simulink model "main"  (R2024b)
settings: Solver=FixedStepAuto  StartTime=0.0  StopTime=2.09  FixedStep=sample_time  RelTol=1e-3
values from neighbouring files (symbols this model uses):
  armTVC = [0 0 0.1064]    [matlab.mat]    (also in vars.m = [)
  att_control_rate = 0.01    [matlab.mat]
  c_d = 0.2    [matlab.mat]    (also in vars.m)
  contact =     [matlab.mat]
  g = 9.807    [matlab.mat]    (also in vars.m)
  initial_euler = [0 0 0]    [matlab.mat]
  m = 0.544    [matlab.mat]    (also in vars.m = 0.472)
  max_angle = 0.13962634016    [matlab.mat]
  rate_control_rate = 0.0025    [matlab.mat]
undefined symbols (not defined in the file or in its folder): fractalcoef, tf_tvc
libraries: sharedtransform x4, aerolibutil x3, sharedutil x3, simulink_extras x2, mspsensorlib x2, uavutilslib x1, shared6dof x1, simulink x1
settings Model: Creator=tommy  LastModifiedBy=tommy

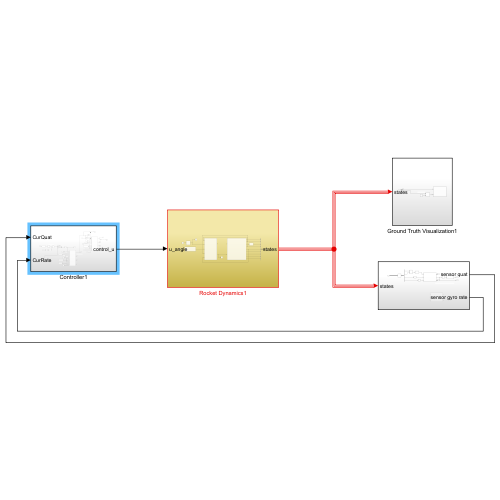
[thumbnail: Simulink's stored preview of the top-level diagram]
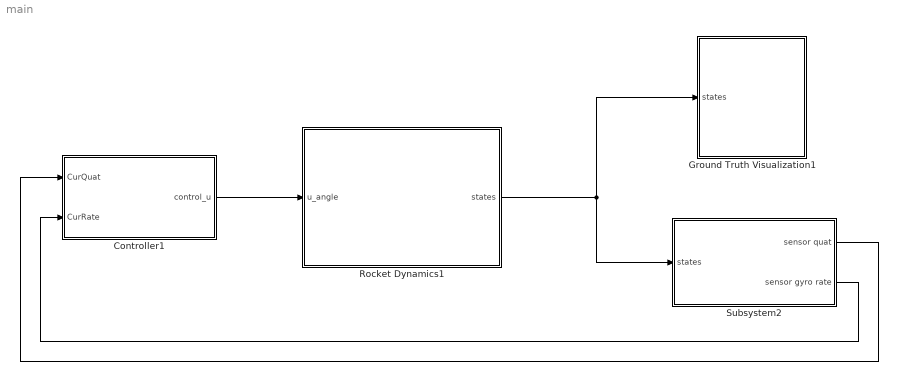
== system main ==
  Controller1 : Subsystem
  Ground Truth Visualization1 : Subsystem
  Rocket Dynamics1 : Subsystem
  Subsystem2 : Subsystem
  wires:
  Subsystem2/2(sensor gyro rate) -> Controller1/2(CurRate)
  Controller1/1(control_u) -> Rocket Dynamics1/1(u_angle)
  Subsystem2/1(sensor quat) -> Controller1/1(CurQuat)
  Rocket Dynamics1/1(states) -> Subsystem2/1(states), Ground Truth Visualization1/1(states)

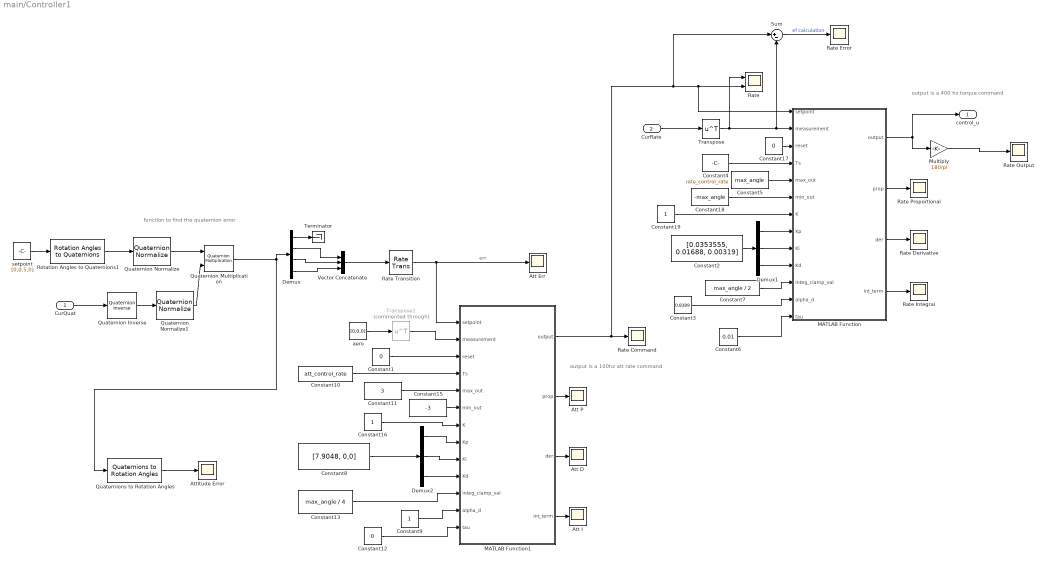
== system main/Controller1 ==
  note: output is a 100hz att rate command
  note: function to find the quaternion error
  note: output is a 400 hz torque command
  CurQuat : Inport
  CurRate : Inport  Port=2
  Att D : Scope
  Att Err : Scope
  Att I : Scope
  Att P : Scope
  Attitude Error : Scope
  Constant1 : Constant  Value=0
  Constant10 : Constant  Value=att_control_rate
  Constant11 : Constant  Value=3
  Constant12 : Constant  Value=0
  Constant13 : Constant  Value=max_angle / 4
  Constant15 : Constant  Value=-3
  Constant16 : Constant
  Constant17 : Constant  Value=0
  Constant18 : Constant  Value=-max_angle
  Constant19 : Constant
  Constant2 : Constant  Value=[0.0353555, 0.01688, 0.00319]
  Constant3 : Constant  Value=0.8389
  Constant4 : Constant  Value=rate_control_rate
  Constant5 : Constant  Value=max_angle
  Constant6 : Constant  Value=0.01
  Constant7 : Constant  Value=max_angle / 2
  Constant8 : Constant  Value=[7.9048, 0,0]
  Constant9 : Constant
  Demux : Demux
  Demux1 : Demux  Outputs=3
  Demux2 : Demux  Outputs=3
  MATLAB Function : MATLAB Function  TreatAsAtomicUnit=on  SystemSampleTime=rate_control_rate
  MATLAB Function1 : MATLAB Function  TreatAsAtomicUnit=on  SystemSampleTime=att_control_rate
  Multiply : Gain  Gain=180/pi
  Quaternion Inverse : aerolibutil/Quaternion Inverse
  Quaternion Multiplication : aerolibutil/Quaternion Multiplication
  Quaternion Normalize : sharedutil/Quaternion Normalize  aMode=aMode
  Quaternion Normalize1 : sharedutil/Quaternion Normalize  aMode=aMode
  Quaternions to Rotation Angles : sharedtransform/Quaternions to Rotation Angles  rotationOrder=XYZ  aMode=aMode
  Rate : Scope  NumInputPorts=2
  Rate Command : Scope
  Rate Derivative : Scope
  Rate Error : Scope
  Rate Integral : Scope
  Rate Output : Scope
  Rate Proportional : Scope
  Rate Transition : RateTransition  OutPortSampleTime=att_control_rate
  Rotation Angles to Quaternions1 : sharedtransform/Rotation Angles to Quaternions  rotationOrder=XYZ  aMode=aMode
  Sum : Sum  Inputs=|+-
  Terminator : Terminator
  Transpose : Math  Operator=transpose
  Transpose1 : Math  Commented=through  Operator=transpose
  Vector Concatenate : Concatenate  NumInputs=3
  aero : Constant  Value=[0,0,0]
  setpoint : Constant  Value=[0,0.5,0]
  control_u : Outport
  wires:
  setpoint/1 -> Rotation Angles to Quaternions1/1
  CurQuat/1 -> Quaternion Inverse/1
  Rotation Angles to Quaternions1/1 -> Quaternion Normalize/1
  Quaternion Inverse/1 -> Quaternion Normalize1/1
  Quaternion Normalize/1 -> Quaternion Multiplication/1
  Quaternion Normalize1/1 -> Quaternion Multiplication/2
  Demux/1 -> Terminator/1
  Quaternion Multiplication/1 -> Demux/1, Quaternions to Rotation Angles/1
  Demux/2 -> Vector Concatenate/1
  Demux/3 -> Vector Concatenate/2
  Demux/4 -> Vector Concatenate/3
  Quaternions to Rotation Angles/1 -> Attitude Error/1
  MATLAB Function/1(output) -> control_u/1, Multiply/1
  Vector Concatenate/1 -> Rate Transition/1
  CurRate/1 -> Transpose/1
  Sum/1 -> Rate Error/1  "ef calculation"
  Constant4/1 -> MATLAB Function/4(Ts)
  Transpose/1 -> MATLAB Function/2(measurement), Sum/2, Rate/1
  Constant6/1 -> MATLAB Function/13(tau)
  MATLAB Function/4(int_term) -> Rate Integral/1
  MATLAB Function/3(der) -> Rate Derivative/1
  MATLAB Function/2(prop) -> Rate Proportional/1
  Constant8/1 -> Demux2/1
  aero/1 -> Transpose1/1
  MATLAB Function1/2(prop) -> Att P/1
  MATLAB Function1/3(der) -> Att D/1
  MATLAB Function1/4(int_term) -> Att I/1
  Rate Transition/1 -> MATLAB Function1/1(setpoint), Att Err/1  "err"
  Demux2/1 -> MATLAB Function1/8(Kp)
  Demux2/2 -> MATLAB Function1/9(Ki)
  Demux2/3 -> MATLAB Function1/10(Kd)
  Constant13/1 -> MATLAB Function1/11(integ_clamp_val)
  Constant9/1 -> MATLAB Function1/12(alpha_d)
  Constant12/1 -> MATLAB Function1/13(tau)
  Constant10/1 -> MATLAB Function1/4(Ts)
  Constant1/1 -> MATLAB Function1/3(reset)
  Constant11/1 -> MATLAB Function1/5(max_out)
  Constant15/1 -> MATLAB Function1/6(min_out)
  Constant16/1 -> MATLAB Function1/7(K)
  Constant17/1 -> MATLAB Function/3(reset)
  Constant2/1 -> Demux1/1
  Constant3/1 -> MATLAB Function/12(alpha_d)
  Constant5/1 -> MATLAB Function/5(max_out)
  Constant18/1 -> MATLAB Function/6(min_out)
  Constant7/1 -> MATLAB Function/11(integ_clamp_val)
  Demux1/3 -> MATLAB Function/10(Kd)
  Demux1/2 -> MATLAB Function/9(Ki)
  Demux1/1 -> MATLAB Function/8(Kp)
  Constant19/1 -> MATLAB Function/7(K)
  Multiply/1 -> Rate Output/1
  Transpose1/1 -> MATLAB Function1/2(measurement)
  MATLAB Function1/1(output) -> Sum/1, MATLAB Function/1(setpoint), Rate/2, Rate Command/1

== system main/Ground Truth Visualization1 ==
  note: orient facing upwards
  states : Inport
  Bus Selector : BusSelector  OutputSignals=Xe,quat
  Constant : Constant  Value=eul2quat([0, pi/2, 0])  VectorParams1D=off
  Quaternion Multiplication : aerolibutil/Quaternion Multiplication
  UAV Animation1 : uavutilslib/UAV Animation  NumUAV=1  DynamicUAVConfig=off  UAVType=FixedWing  UAVSize=1  UAVColor=[1 0 0]  UAVTrajectoryAlpha=1  InertialZDirection=Down  RotationFormat=Quaternion  DrawMarkers=off  SampleTime=0.01
  wires:
  Constant/1 -> Quaternion Multiplication/2
  Quaternion Multiplication/1 -> UAV Animation1/2
  states/1 -> Bus Selector/1
  Bus Selector/1 -> UAV Animation1/1  "<Xe>"
  Bus Selector/2 -> Quaternion Multiplication/1  "<quat>"

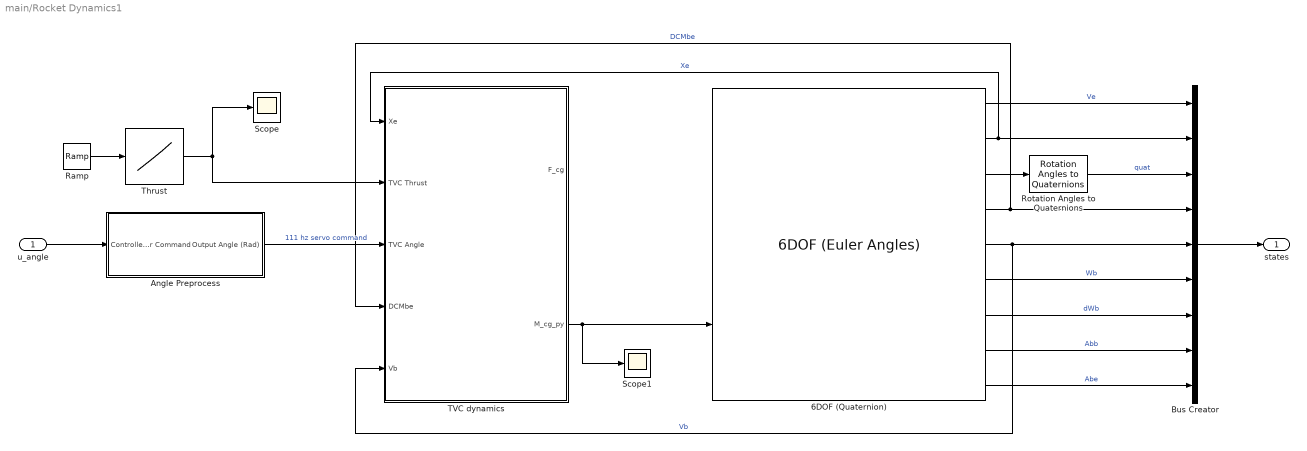
== system main/Rocket Dynamics1 ==
  u_angle : Inport
  6DOF (Quaternion) : shared6dof/6DOF (Euler Angles)  units=Metric (MKS)  mtype=Fixed  rep=Quaternion  xme_0=[0 0 0]  Vm_0=[0 0 0]  eul_0=initial_euler  pm_0=[0 0 0]  mass_0=m  mass_e=0.5  mass_f=2.0  inertia=inertia  inertia_e=eye(3)  inertia_f=2*eye(3)  k_quat=1  vre_flag=on  abi_flag=on  aMode=0  xme_statename=''  Vm_statename=''  eul_statename=''  quat_statename=''  pm_statename=''  mass_statename=''
  Angle Preprocess : Subsystem
  Bus Creator : BusCreator  Inputs=9
  Ramp : simulink/Sources/Ramp  slope=1  start=0  InitialOutput=0
  Rotation Angles to Quaternions : sharedtransform/Rotation Angles to Quaternions  rotationOrder=XYZ  aMode=aMode
  Scope : Scope
  Scope1 : Scope
  TVC dynamics : Subsystem
  Thrust : Lookup_n-D  NumberOfTableDimensions=1  BreakpointsForDimension1=[0;0.15;0.186;0.206;0.242;0.252;0.277;0.333;0.359;0.374;0.394;0.435;0.476;0.521;0.643;0.725;0.821;0.898;1.025;1.142;1.259;1.396;1.569;1.757;1.895;2.027;2.042;2.052;2.063;2.09;4;10]  Table=[0;1.371;1.92;3.387;5.587;7.422;8.705;13.474;15.858;16.592;18.609;21.544;24.661;26.44;21.72;20.432;19.511;18.958;18.219;18.032;17.844;17.472;17.282;17.275;17.086;17.816;12.494;8.457;4.97;0;0;0]  InterpMethod=Akima spline  InternalRulePriority=Speed  RndMeth=Simplest
  states : Outport
  wires:
  Bus Creator/1 -> states/1
  TVC dynamics/2(M_cg_py) -> Scope1/1, 6DOF (Quaternion)/2
  6DOF (Quaternion)/7 -> Bus Creator/7  "dWb"
  Angle Preprocess/1(Output Angle (Rad)) -> TVC dynamics/3(TVC Angle)  "111 hz servo command"
  6DOF (Quaternion)/3 -> Rotation Angles to Quaternions/1
  6DOF (Quaternion)/6 -> Bus Creator/6  "Wb"
  6DOF (Quaternion)/9 -> Bus Creator/9  "Abe"
  6DOF (Quaternion)/5 -> TVC dynamics/5(Vb), Bus Creator/5  "Vb"
  6DOF (Quaternion)/1 -> Bus Creator/1  "Ve"
  u_angle/1 -> Angle Preprocess/1(Controller Command)
  6DOF (Quaternion)/4 -> TVC dynamics/4(DCMbe), Bus Creator/4  "DCMbe"
  6DOF (Quaternion)/2 -> TVC dynamics/1(Xe), Bus Creator/2  "Xe"
  Rotation Angles to Quaternions/1 -> Bus Creator/3  "quat"
  Thrust/1 -> TVC dynamics/2(TVC Thrust), Scope/1
  Ramp/1 -> Thrust/1
  6DOF (Quaternion)/8 -> Bus Creator/8  "Abb"

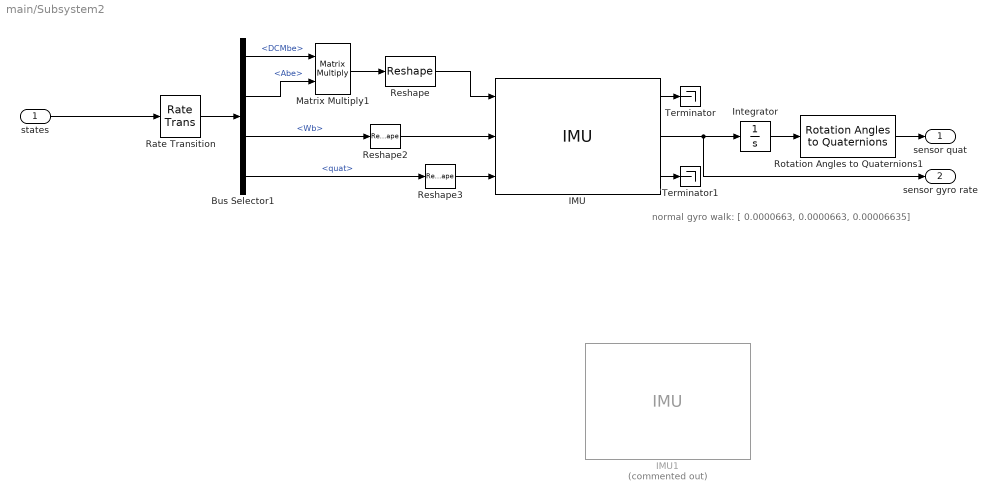
== system main/Subsystem2 ==
  note: normal gyro walk: [ 0.0000663, 0.0000663, 0.00006635]
  states : Inport
  Bus Selector1 : BusSelector  OutputSignals=DCMbe,Abe,Wb,quat
  IMU : mspsensorlib/IMU  DispRefFrame=NED  TemperaturePort=off  Temperature=0  MagneticFieldPort=off  MagneticFieldNED=[ 27.5550, -2.4169, -16.0849 ]  MagneticFieldENU=[ -2.4169, 27.5550, 16.0849 ]  SeedDouble=67  SimulateUsing=Interpreted execution  AccelParamsMeasurementRange=Inf  AccelParamsResolution=0  AccelParamsConstantBias=[ 0, 0, 0 ]  AccelParamsAxesMisalignment=[ 1, 0, 0; 0, 1, 0; 0, 0, 1 ]  AccelParamsNoiseDensity=[ 0, 0, 0 ]  AccelParamsBiasInstability=[ 0, 0, 0 ]  AccelParamsBiasInstabilityNumerator=fractalcoef().Numerator  AccelParamsBiasInstabilityDenominator=fractalcoef().Denominator  AccelParamsRandomWalk=[ 0, 0, 0 ]  AccelParamsNoiseType=double-sided  AccelParamsTemperatureBias=[ 0, 0, 0 ]  AccelParamsTemperatureScaleFactor=[ 0, 0, 0 ]  GyroParamsMeasurementRange=Inf  GyroParamsResolution=0  GyroParamsConstantBias=[ 0, 0, 0 ]  GyroParamsAxesMisalignment=[ 100, 0, 0; 0, 100, 0; 0, 0, 100 ]  GyroParamsAccelerationBias=[ 0, 0, 0 ]  GyroParamsNoiseDensity=[0, 0, 0]  GyroParamsBiasInstability=[ 0, 0, 0 ]  GyroParamsBiasInstabilityNumerator=fractalcoef().Numerator  GyroParamsBiasInstabilityDenominator=fractalcoef().Denominator  GyroParamsRandomWalk=[ 0, 0, 0 ]  GyroParamsNoiseType=double-sided  GyroParamsTemperatureBias=[ 0, 0, 0 ]  GyroParamsTemperatureScaleFactor=[ 0, 0, 0 ]  MagParamsMeasurementRange=Inf  MagParamsResolution=0  MagParamsConstantBias=[ 0, 0, 0 ]  MagParamsAxesMisalignment=[ 100, 0, 0; 0, 100, 0; 0, 0, 100 ]  MagParamsNoiseDensity=[ 0, 0, 0 ]  MagParamsBiasInstability=[ 0, 0, 0 ]  MagParamsBiasInstabilityNumerator=fractalcoef().Numerator  MagParamsBiasInstabilityDenominator=fractalcoef().Denominator  MagParamsRandomWalk=[ 0, 0, 0 ]  MagParamsNoiseType=double-sided  MagParamsTemperatureBias=[ 0, 0, 0 ]  MagParamsTemperatureScaleFactor=[ 0, 0, 0 ]
  IMU1 : mspsensorlib/IMU  Commented=on  DispRefFrame=NED  TemperaturePort=off  Temperature=0  MagneticFieldPort=off  MagneticFieldNED=[ 27.5550, -2.4169, -16.0849 ]  MagneticFieldENU=[ -2.4169, 27.5550, 16.0849 ]  SeedDouble=67  SimulateUsing=Interpreted execution  AccelParamsMeasurementRange=Inf  AccelParamsResolution=0  AccelParamsConstantBias=[ 0, 0, 0 ]  AccelParamsAxesMisalignment=[ 1, 0, 0; 0, 1, 0; 0, 0, 1 ]  AccelParamsNoiseDensity=[ 0, 0, 0 ]  AccelParamsBiasInstability=[ 0, 0, 0 ]  AccelParamsBiasInstabilityNumerator=fractalcoef().Numerator  AccelParamsBiasInstabilityDenominator=fractalcoef().Denominator  AccelParamsRandomWalk=[ 0, 0, 0 ]  AccelParamsNoiseType=double-sided  AccelParamsTemperatureBias=[ 0, 0, 0 ]  AccelParamsTemperatureScaleFactor=[ 0, 0, 0 ]  GyroParamsMeasurementRange=Inf  GyroParamsResolution=0  GyroParamsConstantBias=[ 0, 0, 0 ]  GyroParamsAxesMisalignment=[ 100, 0, 0; 0, 100, 0; 0, 0, 100 ]  GyroParamsAccelerationBias=[ 0, 0, 0 ]  GyroParamsNoiseDensity=[ 0.0000663, 0.0000663, 0.00006635]  GyroParamsBiasInstability=[ 0, 0, 0 ]  GyroParamsBiasInstabilityNumerator=fractalcoef().Numerator  GyroParamsBiasInstabilityDenominator=fractalcoef().Denominator  GyroParamsRandomWalk=[ 0, 0, 0 ]  GyroParamsNoiseType=double-sided  GyroParamsTemperatureBias=[ 0, 0, 0 ]  GyroParamsTemperatureScaleFactor=[ 0, 0, 0 ]  MagParamsMeasurementRange=Inf  MagParamsResolution=0  MagParamsConstantBias=[ 0, 0, 0 ]  MagParamsAxesMisalignment=[ 100, 0, 0; 0, 100, 0; 0, 0, 100 ]  MagParamsNoiseDensity=[ 0, 0, 0 ]  MagParamsBiasInstability=[ 0, 0, 0 ]  MagParamsBiasInstabilityNumerator=fractalcoef().Numerator  MagParamsBiasInstabilityDenominator=fractalcoef().Denominator  MagParamsRandomWalk=[ 0, 0, 0 ]  MagParamsNoiseType=double-sided  MagParamsTemperatureBias=[ 0, 0, 0 ]  MagParamsTemperatureScaleFactor=[ 0, 0, 0 ]
  Integrator : Integrator  InitialCondition=initial_euler
  Matrix Multiply1 : Product  Multiplication=Matrix(*)
  Rate Transition : RateTransition  OutPortSampleTime=sample_time
  Reshape : Reshape  OutputDimensionality=Row vector (2-D)
  Reshape2 : Reshape  OutputDimensionality=Row vector (2-D)
  Reshape3 : Reshape  OutputDimensionality=Row vector (2-D)
  Rotation Angles to Quaternions1 : sharedtransform/Rotation Angles to Quaternions  rotationOrder=XYZ  aMode=aMode
  Terminator : Terminator
  Terminator1 : Terminator
  sensor quat : Outport
  sensor gyro rate : Outport  Port=2
  wires:
  Reshape2/1 -> IMU/2
  IMU/2 -> Integrator/1, sensor gyro rate/1
  Matrix Multiply1/1 -> Reshape/1
  Reshape/1 -> IMU/1
  Integrator/1 -> Rotation Angles to Quaternions1/1
  Reshape3/1 -> IMU/3
  Bus Selector1/4 -> Reshape3/1  "<quat>"
  Bus Selector1/3 -> Reshape2/1  "<Wb>"
  Rotation Angles to Quaternions1/1 -> sensor quat/1
  states/1 -> Rate Transition/1
  Rate Transition/1 -> Bus Selector1/1
  IMU/1 -> Terminator/1
  IMU/3 -> Terminator1/1
  Bus Selector1/1 -> Matrix Multiply1/1  "<DCMbe>"
  Bus Selector1/2 -> Matrix Multiply1/2  "<Abe>"

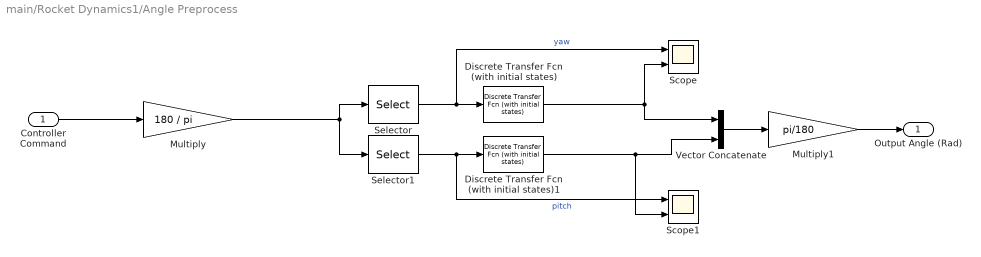
== system main/Rocket Dynamics1/Angle Preprocess ==
  Controller Command : Inport
  Discrete Transfer Fcn (with initial states) : simulink_extras/Additional Discrete/Discrete Transfer Fcn (with initial states)  N=tf_tvc.Numerator  D=tf_tvc.Denominator  X0=[1]  TS=tf_tvc.Ts
  Discrete Transfer Fcn (with initial states)1 : simulink_extras/Additional Discrete/Discrete Transfer Fcn (with initial states)  N=tf_tvc.Numerator  D=tf_tvc.Denominator  X0=[1]  TS=tf_tvc.Ts
  Multiply : Gain  Gain=180 / pi
  Multiply1 : Gain  Gain=pi/180
  Scope : Scope  NumInputPorts=2
  Scope1 : Scope  NumInputPorts=2
  Selector : Selector  InputPortWidth=3  IndexOptions=Index vector (dialog)  Indices=[1]  OutputSizes=1
  Selector1 : Selector  InputPortWidth=3  IndexOptions=Index vector (dialog)  Indices=[2]  OutputSizes=1
  Vector Concatenate : Concatenate
  Output Angle (Rad) : Outport
  wires:
  Vector Concatenate/1 -> Multiply1/1
  Controller Command/1 -> Multiply/1
  Selector/1 -> Discrete Transfer Fcn (with initial states)/1, Scope/1  "yaw"
  Multiply1/1 -> Output Angle (Rad)/1
  Discrete Transfer Fcn (with initial states)/1 -> Vector Concatenate/1, Scope/2
  Discrete Transfer Fcn (with initial states)1/1 -> Scope1/2, Vector Concatenate/2
  Multiply/1 -> Selector1/1, Selector/1
  Selector1/1 -> Scope1/1, Discrete Transfer Fcn (with initial states)1/1  "pitch"

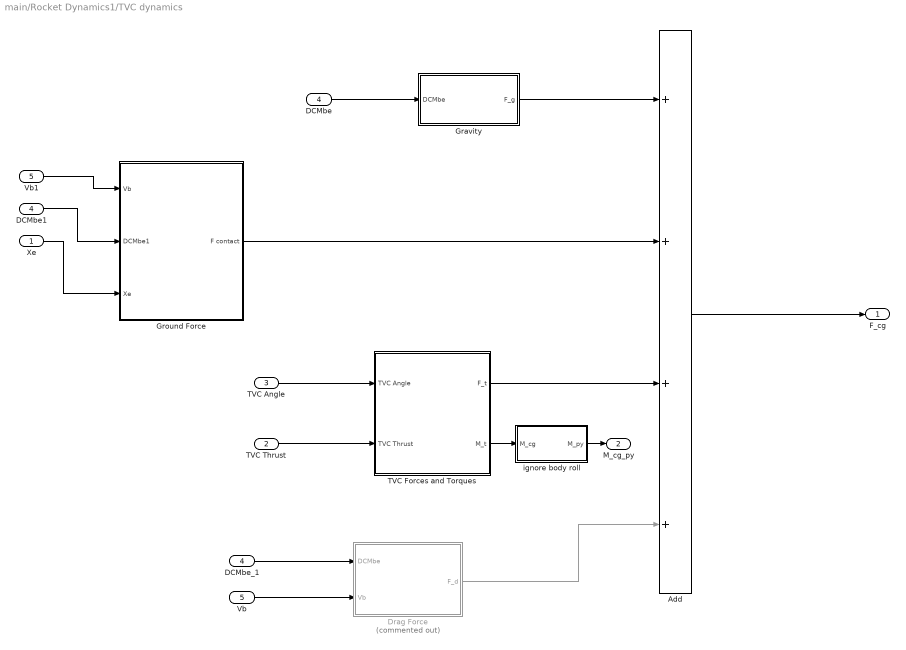
== system main/Rocket Dynamics1/TVC dynamics ==
  Xe : Inport
  TVC Thrust : Inport  Port=2
  TVC Angle : Inport  Port=3
  DCMbe : Inport  Port=4
  Vb : Inport  Port=5
  Add : Sum  Inputs=++++
  DCMbe1 : InportShadow  Port=4
  DCMbe_1 : InportShadow  Port=4
  Drag Force : Subsystem  Commented=on
  Gravity : Subsystem
  Ground Force : Subsystem
  TVC Forces and Torques : Subsystem
  Vb1 : InportShadow  Port=5
  "ignore body roll " : Subsystem
  F_cg : Outport
  M_cg_py : Outport  Port=2
  wires:
  Add/1 -> F_cg/1
  DCMbe_1/1 -> Drag Force/1(DCMbe)
  TVC Forces and Torques/1(F_t) -> Add/3
  Vb/1 -> Drag Force/2(Vb)
  Gravity/1(F_g) -> Add/1
  TVC Thrust/1 -> TVC Forces and Torques/2(TVC Thrust)
  TVC Forces and Torques/2(M_t) -> "ignore body roll "/1(M_cg)
  DCMbe/1 -> Gravity/1(DCMbe)
  TVC Angle/1 -> TVC Forces and Torques/1(TVC Angle)
  Drag Force/1(F_d) -> Add/4
  DCMbe1/1 -> Ground Force/2(DCMbe1)
  Xe/1 -> Ground Force/3(Xe)
  Ground Force/1(F contact) -> Add/2
  Vb1/1 -> Ground Force/1(Vb)
  "ignore body roll "/1(M_py) -> M_cg_py/1

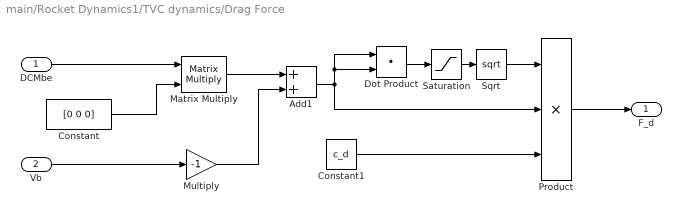
== system main/Rocket Dynamics1/TVC dynamics/Drag Force ==
  DCMbe : Inport
  Vb : Inport  Port=2
  Add1 : Sum
  Constant : Constant  Value=[0 0 0]
  Constant1 : Constant  Value=c_d
  Dot Product : DotProduct  OutDataTypeStr=Inherit: Inherit via internal rule
  Matrix Multiply : Product  Multiplication=Matrix(*)
  Multiply : Gain  Gain=-1
  Product : Product  Inputs=3
  Saturation : Saturate  UpperLimit=inf  LowerLimit=0.00001
  Sqrt : Sqrt
  F_d : Outport
  wires:
  Dot Product/1 -> Saturation/1
  Multiply/1 -> Add1/2
  Constant/1 -> Matrix Multiply/2
  Matrix Multiply/1 -> Add1/1
  Add1/1 -> Product/2, Dot Product/1, Dot Product/2
  Vb/1 -> Multiply/1
  DCMbe/1 -> Matrix Multiply/1
  Sqrt/1 -> Product/1
  Saturation/1 -> Sqrt/1
  Product/1 -> F_d/1
  Constant1/1 -> Product/3

== system main/Rocket Dynamics1/TVC dynamics/Gravity ==
  DCMbe : Inport
  Constant : Constant  Value=[0 0 g]
  Matrix Multiply : Product  Multiplication=Matrix(*)
  Multiply : Gain  Gain=m
  F_g : Outport
  wires:
  Multiply/1 -> Matrix Multiply/2
  DCMbe/1 -> Matrix Multiply/1
  Constant/1 -> Multiply/1
  Matrix Multiply/1 -> F_g/1

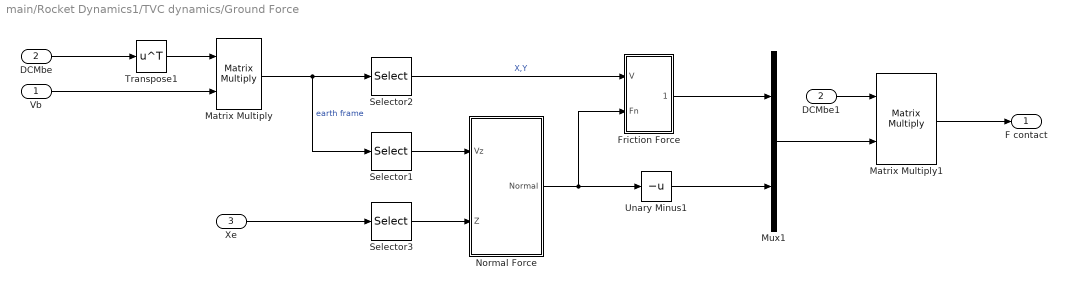
== system main/Rocket Dynamics1/TVC dynamics/Ground Force ==
  Vb : Inport
  DCMbe1 : Inport  Port=2
  Xe : Inport  Port=3
  DCMbe : InportShadow  Port=2
  Friction Force : Subsystem
  Matrix Multiply : Product  Multiplication=Matrix(*)
  Matrix Multiply1 : Product  Multiplication=Matrix(*)
  Mux1 : Mux  Inputs=2
  Normal Force : Subsystem
  Selector1 : Selector  InputPortWidth=3  IndexOptions=Index vector (dialog)  Indices=[3]  OutputSizes=1
  Selector2 : Selector  InputPortWidth=3  IndexOptions=Index vector (dialog)  Indices=[1,2]  OutputSizes=1
  Selector3 : Selector  InputPortWidth=3  IndexOptions=Index vector (dialog)  Indices=[3]  OutputSizes=1
  Transpose1 : Math  Operator=transpose
  Unary Minus1 : UnaryMinus
  F contact : Outport
  wires:
  Matrix Multiply1/1 -> F contact/1
  Friction Force/1(Friction) -> Mux1/1
  Xe/1 -> Selector3/1
  Vb/1 -> Matrix Multiply/2
  Selector3/1 -> Normal Force/2(Z)
  Matrix Multiply/1 -> Selector1/1, Selector2/1  "earth frame"
  Mux1/1 -> Matrix Multiply1/2
  Selector2/1 -> Friction Force/1(V)  "X,Y"
  Selector1/1 -> Normal Force/1(Vz)
  DCMbe1/1 -> Matrix Multiply1/1
  DCMbe/1 -> Transpose1/1
  Transpose1/1 -> Matrix Multiply/1
  Unary Minus1/1 -> Mux1/2
  Normal Force/1(Normal) -> Unary Minus1/1, Friction Force/2(Fn)

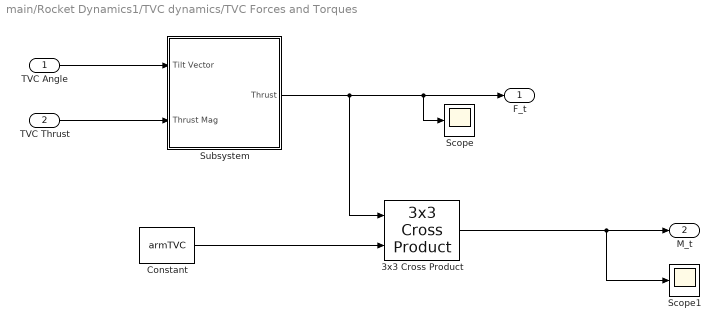
== system main/Rocket Dynamics1/TVC dynamics/TVC Forces and Torques ==
  TVC Angle : Inport
  TVC Thrust : Inport  Port=2
  3x3 Cross Product : sharedutil/3x3 Cross Product  aMode=aMode
  Constant : Constant  Value=armTVC
  Scope : Scope
  Scope1 : Scope
  Subsystem : Subsystem
  F_t : Outport
  M_t : Outport  Port=2
  wires:
  TVC Angle/1 -> Subsystem/1(Tilt Vector)
  TVC Thrust/1 -> Subsystem/2(Thrust Mag)
  Subsystem/1(Thrust) -> 3x3 Cross Product/1, Scope/1, F_t/1
  Constant/1 -> 3x3 Cross Product/2
  3x3 Cross Product/1 -> Scope1/1, M_t/1

== system main/Rocket Dynamics1/TVC dynamics/ignore body roll  ==
  M_cg : Inport
  Constant1 : Constant  Value=[1, 1, 0]
  Matrix Multiply : Product
  M_py : Outport
  wires:
  Constant1/1 -> Matrix Multiply/1
  Matrix Multiply/1 -> M_py/1
  M_cg/1 -> Matrix Multiply/2

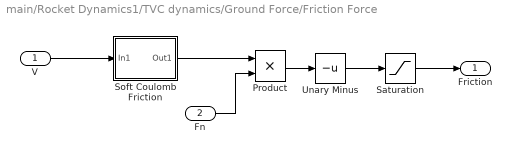
== system main/Rocket Dynamics1/TVC dynamics/Ground Force/Friction Force ==
  V : Inport
  Fn : Inport  Port=2
  Product : Product
  Saturation : Saturate  UpperLimit=contact.translation.maxFriction  LowerLimit=-contact.translation.maxFriction
  Soft Coulomb Friction : Subsystem
  Unary Minus : UnaryMinus
  Friction : Outport
  wires:
  Fn/1 -> Product/2
  Soft Coulomb Friction/1(Out1) -> Product/1
  Product/1 -> Unary Minus/1
  V/1 -> Soft Coulomb Friction/1(In1)
  Unary Minus/1 -> Saturation/1
  Saturation/1 -> Friction/1

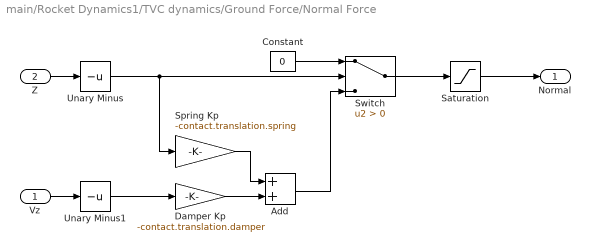
== system main/Rocket Dynamics1/TVC dynamics/Ground Force/Normal Force ==
  Vz : Inport
  Z : Inport  Port=2
  Add : Sum
  Constant : Constant  Value=0
  Damper Kp : Gain  Gain=-contact.translation.damper
  Saturation : Saturate  UpperLimit=contact.translation.maxNormal  LowerLimit=0
  Spring Kp : Gain  Gain=-contact.translation.spring
  Switch : Switch  Criteria=u2 > Threshold  SaturateOnIntegerOverflow=off  InputSameDT=off
  Unary Minus : UnaryMinus
  Unary Minus1 : UnaryMinus
  Normal : Outport
  wires:
  Constant/1 -> Switch/1
  Z/1 -> Unary Minus/1
  Switch/1 -> Saturation/1
  Damper Kp/1 -> Add/2
  Add/1 -> Switch/3
  Spring Kp/1 -> Add/1
  Vz/1 -> Unary Minus1/1
  Saturation/1 -> Normal/1
  Unary Minus/1 -> Spring Kp/1, Switch/2
  Unary Minus1/1 -> Damper Kp/1

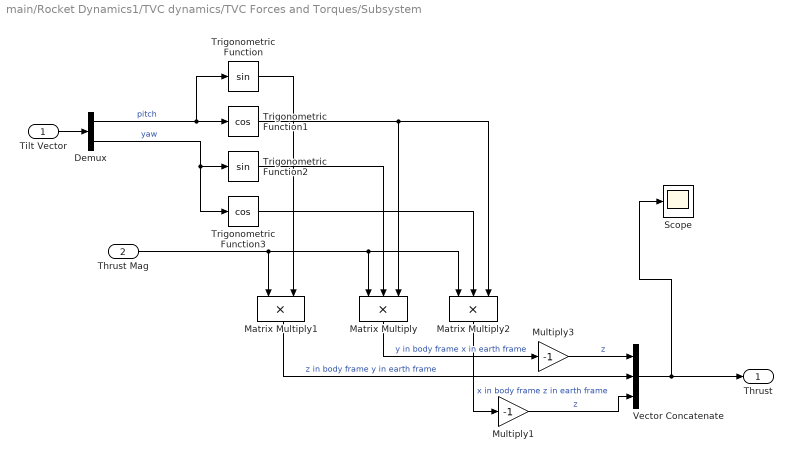
== system main/Rocket Dynamics1/TVC dynamics/TVC Forces and Torques/Subsystem ==
  Tilt Vector : Inport
  Thrust Mag : Inport  Port=2
  Demux : Demux  Outputs=2
  Matrix Multiply : Product  Inputs=3
  Matrix Multiply1 : Product
  Matrix Multiply2 : Product  Inputs=3
  Multiply1 : Gain  Gain=-1
  Multiply3 : Gain  Gain=-1
  Scope : Scope
  Trigonometric Function : Trigonometry
  Trigonometric Function1 : Trigonometry  Operator=cos
  Trigonometric Function2 : Trigonometry
  Trigonometric Function3 : Trigonometry  Operator=cos
  Vector Concatenate : Concatenate  NumInputs=3
  Thrust : Outport
  wires:
  Trigonometric Function2/1 -> Matrix Multiply/2
  Demux/2 -> Trigonometric Function3/1, Trigonometric Function2/1  "yaw"
  Matrix Multiply1/1 -> Vector Concatenate/2  "z in body frame y in earth frame"
  Tilt Vector/1 -> Demux/1
  Trigonometric Function1/1 -> Matrix Multiply/3, Matrix Multiply2/3
  Demux/1 -> Trigonometric Function/1, Trigonometric Function1/1  "pitch"
  Trigonometric Function3/1 -> Matrix Multiply2/2
  Thrust Mag/1 -> Matrix Multiply2/1, Matrix Multiply/1, Matrix Multiply1/1
  Vector Concatenate/1 -> Scope/1, Thrust/1
  Trigonometric Function/1 -> Matrix Multiply1/2
  Matrix Multiply2/1 -> Multiply1/1  "x in body frame z in earth frame"
  Multiply1/1 -> Vector Concatenate/3  "z"
  Multiply3/1 -> Vector Concatenate/1  "z"
  Matrix Multiply/1 -> Multiply3/1  "y in body frame x in earth frame"

== system main/Rocket Dynamics1/TVC dynamics/Ground Force/Friction Force/Soft Coulomb Friction ==
  note: Pennestrì, E., Rossi, V., Salvini, P. et al. Review and comparison of dry friction force models. Nonlinear Dyn 83, 1785–1801 (2016). https://doi.org/10.1007/s11071-015-2485-3
  In1 : Inport
  Tanh : Trigonometry  Operator=tanh
  friction coefficient : Gain  Gain=contact.translation.friction
  vd : Gain  Gain=1/contact.translation.vd
  Out1 : Outport
  wires:
  In1/1 -> vd/1
  vd/1 -> Tanh/1
  Tanh/1 -> friction coefficient/1
  friction coefficient/1 -> Out1/1

== matlab function main/Controller1/MATLAB Function ==
  data: setpoint input; output output; prop output; der output; measurement input; reset input; Ts input; max_out input; min_out input; K input; Kp input; Ki input; Kd input; integ_clamp_val input; alpha_d input; tau input; int_term output
function [output, prop, der, int_term] = PID_SF_Matlab(setpoint, measurement, reset, Ts, max_out, min_out, K, Kp, Ki, Kd, integ_clamp_val, alpha_d, tau)
% PID_SF_Matlab: A standard form PID controller translated from a C++ implementation.
%
% This controller features several enhancements over a basic PID:
%   - Derivative on measurement: Prevents "derivative kick" on setpoint changes.
%   - Integral clamping: Directly limits the integral term to prevent excessive windup.
%   - Conditional integration (anti-windup): Stops integration when the output is saturated.
%   - Output filtering: Smooths the final control signal using a low-pass filter.
%
% It is designed to be a "plug-and-play" replacement for the original PID_Simulink
% function and supports N-dimensional vector inputs.
%
% Inputs:
%   setpoint        - Desired setpoint (e.g., 3x1 vector).
%   measurement     - Measured process variable (e.g., 3x1 vector).
%   reset           - Boolean flag (1 or true) to reset the controller's internal states.
%   Ts              - Sampling time in seconds (scalar).
%   max_out         - Maximum output value (scalar).
%   min_out         - Minimum output value (scalar).
%   K               - Overall system gain (scalar).
%   Kp              - Proportional gain (scalar).
%   Ki              - Integral gain (scalar).
%   Kd              - Derivative gain (scalar).
%   integ_clamp_val - User-friendly absolute integral clamp value (e.g., 500 for a servo).
%   alpha_d         - Smoothing factor for the derivative term (0 to 1). A smaller value means more smoothing.
%   tau             - Time constant for the output low-pass filter in seconds (scalar). Larger tau means more smoothing.
%
% Outputs:
%   output          - The final, filtered PID control signal (same dimensions as input).
%   prop            - The proportional component of the output.
%   der             - The derivative component of the output.
%   int_term        - The integral component of the output.

% Declare persistent variables to hold the controller's state between calls.
persistent integral_state prev_meas derivative_state old_output_filtered

% Initialize states to zero on the first call or when the reset flag is true.
% This corrected block ensures persistent variables are only checked with isempty
% before their first assignment.
if isempty(integral_state) || reset
    vec_size = size(setpoint);
    integral_state = zeros(vec_size);
    prev_meas = zeros(vec_size);
    derivative_state = zeros(vec_size);
    old_output_filtered = zeros(vec_size);
end

% --- Parameter Pre-calculation (for efficiency, mirrors C++ setup) ---

% Add robustness against invalid sampling time.
if Ts <= 0
    Ts = 1e-6; % Use a very small number to prevent division by zero.
end

% Pre-multiply/divide gains by Ts to save computation in the main loop.
ki_Ts = Ki * Ts;
kd_Ts = Kd / Ts;

% Scale the user-provided integral clamp value based on the system gains.
% This translates the desired absolute clamp into the correct internal value.
if (K * ki_Ts > 0)
    integ_clamp_scaled = integ_clamp_val / (K * ki_Ts);
else
    integ_clamp_scaled = 0;
end

% Calculate the output low-pass filter coefficient from the time constant.
if (Ts + tau) > 1e-6
    alpha_lpf = Ts / (Ts + tau);
else
    alpha_lpf = 1.0;
end

% --- Core PID Logic ---

% 1. Calculate the error.
error = setpoint - measurement;

% 2. Calculate the filtered derivative on the measurement, not the error.
% This is a low-pass filter on the rate of change of the measurement.
derivative_state = alpha_d .* (measurement - prev_meas) + (1 - alpha_d) .* derivative_state;

% 3. Calculate the individual P, I, and D components for the output signal.
prop     = K .* Kp .* error;
int_term = K .* ki_Ts .* integral_state;
der      = -K .* kd_Ts .* derivative_state; % Note the negative sign.

% 4. Sum the components to get the preliminary, unfiltered output.
output_pre_clamp = prop + int_term + der;

% 5. Apply output saturation and conditional integration (anti-windup).
% This loop is necessary to handle vector inputs correctly.
output = output_pre_clamp;
for i = 1:numel(output)
    if output(i) > max_out
        output(i) = max_out;
    elseif output(i) < min_out
        output(i) = min_out;
    else
        % ONLY update the integral if the output is NOT saturated.
        integral_state(i) = integral_state(i) + error(i);
    end
end

% 6. Apply the direct clamp on the integral state itself.
for i = 1:numel(integral_state)
    if integral_state(i) > integ_clamp_scaled
        integral_state(i) = integ_clamp_scaled;
    elseif integral_state(i) < -integ_clamp_scaled
        integral_state(i) = -integ_clamp_scaled;
    end
end

% 8. Update persistent states for the next function call.
prev_meas = measurement;
old_output_filtered = output;

end

== matlab function main/Controller1/MATLAB Function1 ==
  data: setpoint input; output output; prop output; der output; measurement input; reset input; Ts input; max_out input; min_out input; K input; Kp input; Ki input; Kd input; integ_clamp_val input; alpha_d input; tau input; int_term output
function [output, prop, der, int_term] = PID_SF_Matlab(setpoint, measurement, reset, Ts, max_out, min_out, K, Kp, Ki, Kd, integ_clamp_val, alpha_d, tau)
% PID_SF_Matlab: A standard form PID controller translated from a C++ implementation.
%
% This controller features several enhancements over a basic PID:
%   - Derivative on measurement: Prevents "derivative kick" on setpoint changes.
%   - Integral clamping: Directly limits the integral term to prevent excessive windup.
%   - Conditional integration (anti-windup): Stops integration when the output is saturated.
%   - Output filtering: Smooths the final control signal using a low-pass filter.
%
% It is designed to be a "plug-and-play" replacement for the original PID_Simulink
% function and supports N-dimensional vector inputs.
%
% Inputs:
%   setpoint        - Desired setpoint (e.g., 3x1 vector).
%   measurement     - Measured process variable (e.g., 3x1 vector).
%   reset           - Boolean flag (1 or true) to reset the controller's internal states.
%   Ts              - Sampling time in seconds (scalar).
%   max_out         - Maximum output value (scalar).
%   min_out         - Minimum output value (scalar).
%   K               - Overall system gain (scalar).
%   Kp              - Proportional gain (scalar).
%   Ki              - Integral gain (scalar).
%   Kd              - Derivative gain (scalar).
%   integ_clamp_val - User-friendly absolute integral clamp value (e.g., 500 for a servo).
%   alpha_d         - Smoothing factor for the derivative term (0 to 1). A smaller value means more smoothing.
%   tau             - Time constant for the output low-pass filter in seconds (scalar). Larger tau means more smoothing.
%
% Outputs:
%   output          - The final, filtered PID control signal (same dimensions as input).
%   prop            - The proportional component of the output.
%   der             - The derivative component of the output.
%   int_term        - The integral component of the output.

% Declare persistent variables to hold the controller's state between calls.
persistent integral_state prev_meas derivative_state old_output_filtered

% Initialize states to zero on the first call or when the reset flag is true.
% This corrected block ensures persistent variables are only checked with isempty
% before their first assignment.
if isempty(integral_state) || reset
    vec_size = size(setpoint);
    integral_state = zeros(vec_size);
    prev_meas = zeros(vec_size);
    derivative_state = zeros(vec_size);
    old_output_filtered = zeros(vec_size);
end

% --- Parameter Pre-calculation (for efficiency, mirrors C++ setup) ---

% Add robustness against invalid sampling time.
if Ts <= 0
    Ts = 1e-6; % Use a very small number to prevent division by zero.
end

% Pre-multiply/divide gains by Ts to save computation in the main loop.
ki_Ts = Ki * Ts;
kd_Ts = Kd / Ts;

% Scale the user-provided integral clamp value based on the system gains.
% This translates the desired absolute clamp into the correct internal value.
if (K * ki_Ts > 0)
    integ_clamp_scaled = integ_clamp_val / (K * ki_Ts);
else
    integ_clamp_scaled = 0;
end

% Calculate the output low-pass filter coefficient from the time constant.
if (Ts + tau) > 1e-6
    alpha_lpf = Ts / (Ts + tau);
else
    alpha_lpf = 1.0;
end

% --- Core PID Logic ---

% 1. Calculate the error.
error = setpoint - measurement;

% 2. Calculate the filtered derivative on the measurement, not the error.
% This is a low-pass filter on the rate of change of the measurement.
derivative_state = alpha_d .* (measurement - prev_meas) + (1 - alpha_d) .* derivative_state;

% 3. Calculate the individual P, I, and D components for the output signal.
prop     = K .* Kp .* error;
int_term = K .* ki_Ts .* integral_state;
der      = -K .* kd_Ts .* derivative_state; % Note the negative sign.

% 4. Sum the components to get the preliminary, unfiltered output.
output_pre_clamp = prop + int_term + der;

% 5. Apply output saturation and conditional integration (anti-windup).
% This loop is necessary to handle vector inputs correctly.
output = output_pre_clamp;
for i = 1:numel(output)
    if output(i) > max_out
        output(i) = max_out;
    elseif output(i) < min_out
        output(i) = min_out;
    else
        % ONLY update the integral if the output is NOT saturated.
        integral_state(i) = integral_state(i) + error(i);
    end
end

% 6. Apply the direct clamp on the integral state itself.
for i = 1:numel(integral_state)
    if integral_state(i) > integ_clamp_scaled
        integral_state(i) = integ_clamp_scaled;
    elseif integral_state(i) < -integ_clamp_scaled
        integral_state(i) = -integ_clamp_scaled;
    end
end

% 8. Update persistent states for the next function call.
prev_meas = measurement;
old_output_filtered = output;

end
